simulink library "INT_VehVDspl_DD"  (R2016b)
settings: Solver=VariableStepAuto  StartTime=0.0  StopTime=10.0  RelTol=1e-3
settings Model: Creator=Wei Liang  LastModifiedBy=Wei Liang

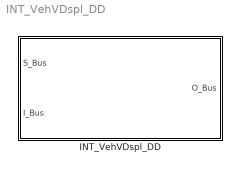
== system INT_VehVDspl_DD ==
  INT_VehVDspl_DD : Subsystem

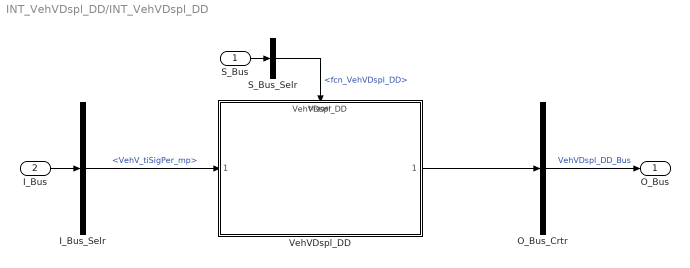
== system INT_VehVDspl_DD/INT_VehVDspl_DD ==
  S_Bus : Inport
  I_Bus : Inport  Port=2
  I_Bus_Selr : BusSelector  OutputSignals=VehV_tiSigPer_mp
  O_Bus_Crtr : BusCreator  Inputs=1
  S_Bus_Selr : BusSelector  OutputSignals=fcn_VehVDspl_DD
  VehVDspl_DD : ModelReference  ModelNameDialog=VehVDspl_DD  SimulationMode=Normal  ModelReferenceVersion=1.5  TriggerPortName=function  TriggerPortTriggerType=function-call  TriggerPortStatesWhenEnabling=held
  O_Bus : Outport
  wires:
  S_Bus_Selr/1 -> VehVDspl_DD/Trigger  "<fcn_VehVDspl_DD>"
  S_Bus/1 -> S_Bus_Selr/1
  I_Bus/1 -> I_Bus_Selr/1
  I_Bus_Selr/1 -> VehVDspl_DD/1  "<VehV_tiSigPer_mp>"
  O_Bus_Crtr/1 -> O_Bus/1  "VehVDspl_DD_Bus"
  VehVDspl_DD/1 -> O_Bus_Crtr/1
